simulink model "c63_cylinder_blowdown_ref"  (R2026a)
settings: Solver=ode4  StopTime=S12_BlowdownStopTimeS  FixedStep=1e-6
model workspace (MAT data in the model file):
  S12_BlowdownStopTimeS = Simulink.Parameter
  S12_BlowdownStopTimeS.Value = 0.0266666666667
  S12_BlowdownStopTimeS.Complexity = 'real'
  S12_BlowdownStopTimeS.Dimensions = [1 1]
  S12_BlowdownStopTimeS.Description = 'Run from -180 to +300 deg ATDC'
  S12_BlowdownStopTimeS.DataType = 'auto'
  S12_BlowdownStopTimeS.DocUnits = 's'
  S12_BurnedCpJkgK = Simulink.Parameter
  S12_BurnedCpJkgK.Value = [1075.46244927 1100.31766319 1127.88587263 1157.95433687 1189.74992272 1221.93910449 1252.627964 1279.36219058 1303.34621886 1325.27401636 1345.29919881 1363.55240895 1380.1594629 1395.24135019 1408.91423372 1421.28944978 1432.47350805 1442.56809158 1451.67005684 1459.87143365 1467.25942525 1473.91640823 1479.91993261 1485.34272177 1490.25267247 1494.71285488 1498.78151253 1502.51206237 1505.9530947 1509.14837323 1512.13683507 1514.95259067 1517.62492391]
  S12_BurnedCpJkgK.Complexity = 'real'
  S12_BurnedCpJkgK.Dimensions = [1 33]
  S12_BurnedCpJkgK.Description = 'Derived from NASA species polynomial mixture tables'
  S12_BurnedCpJkgK.DataType = 'auto'
  S12_BurnedCpJkgK.DocUnits = 'J/(kg*K)'
  S12_BurnedGasConstantJkgK = Simulink.Parameter
  S12_BurnedGasConstantJkgK.Value = 290.645082378
  S12_BurnedGasConstantJkgK.Complexity = 'real'
  S12_BurnedGasConstantJkgK.Dimensions = [1 1]
  S12_BurnedGasConstantJkgK.Description = 'Derived from NASA species polynomial mixture tables'
  S12_BurnedGasConstantJkgK.DataType = 'auto'
  S12_BurnedGasConstantJkgK.DocUnits = 'J/(kg*K)'
  S12_C63_BoreM = Simulink.Parameter
  S12_C63_BoreM.Value = 0.1022
  S12_C63_BoreM.Complexity = 'real'
  S12_C63_BoreM.Dimensions = [1 1]
  S12_C63_BoreM.Description = 'Grade A M156.985 bore'
  S12_C63_BoreM.DataType = 'auto'
  S12_C63_BoreM.DocUnits = 'm'
  S12_C63_CompressionRatio = Simulink.Parameter
  S12_C63_CompressionRatio.Value = 11.3
  S12_C63_CompressionRatio.Complexity = 'real'
  S12_C63_CompressionRatio.Dimensions = [1 1]
  S12_C63_CompressionRatio.Description = 'Grade A M156.985 compression ratio'
  S12_C63_CompressionRatio.DataType = 'auto'
  S12_C63_RodLengthM = Simulink.Parameter
  S12_C63_RodLengthM.Value = 0.1455
  S12_C63_RodLengthM.Complexity = 'real'
  S12_C63_RodLengthM.Dimensions = [1 1]
  S12_C63_RodLengthM.Description = 'Grade D identification initial value'
  S12_C63_RodLengthM.DataType = 'auto'
  S12_C63_RodLengthM.DocUnits = 'm'
  S12_C63_StrokeM = Simulink.Parameter
  S12_C63_StrokeM.Value = 0.0946
  S12_C63_StrokeM.Complexity = 'real'
  S12_C63_StrokeM.Dimensions = [1 1]
  S12_C63_StrokeM.Description = 'Grade A M156.985 stroke'
  S12_C63_StrokeM.DataType = 'auto'
  S12_C63_StrokeM.DocUnits = 'm'
  S12_CrankDegPerSecond = Simulink.Parameter
  S12_CrankDegPerSecond.Value = 18000
  S12_CrankDegPerSecond.Complexity = 'real'
  S12_CrankDegPerSecond.Dimensions = [1 1]
  S12_CrankDegPerSecond.Description = 'Derived crank speed'
  S12_CrankDegPerSecond.DataType = 'auto'
  S12_CrankDegPerSecond.DocUnits = 'deg/s'
  S12_DownstreamPressurePa = Simulink.Parameter
  S12_DownstreamPressurePa.Value = 101325
  S12_DownstreamPressurePa.Complexity = 'real'
  S12_DownstreamPressurePa.Dimensions = [1 1]
  S12_DownstreamPressurePa.Description = 'Reference exhaust manifold pressure'
  S12_DownstreamPressurePa.DataType = 'auto'
  S12_DownstreamPressurePa.DocUnits = 'Pa'
  S12_EngineRPM = Simulink.Parameter
  S12_EngineRPM.Value = 3000
  S12_EngineRPM.Complexity = 'real'
  S12_EngineRPM.Dimensions = [1 1]
  S12_EngineRPM.Description = 'Reference operating point'
  S12_EngineRPM.DataType = 'auto'
  S12_EngineRPM.DocUnits = 'rpm'
  S12_EvoDegATDC = Simulink.Parameter
  S12_EvoDegATDC.Value = 130
  S12_EvoDegATDC.Complexity = 'real'
  S12_EvoDegATDC.Dimensions = [1 1]
  S12_EvoDegATDC.Description = 'Grade D EVO initial value'
  S12_EvoDegATDC.DataType = 'auto'
  S12_EvoDegATDC.DocUnits = 'deg'
  S12_ExhaustDurationDeg = Simulink.Parameter
  S12_ExhaustDurationDeg.Value = 220
  S12_ExhaustDurationDeg.Complexity = 'real'
  S12_ExhaustDurationDeg.Dimensions = [1 1]
  S12_ExhaustDurationDeg.Description = 'Grade D exhaust duration'
  S12_ExhaustDurationDeg.DataType = 'auto'
  S12_ExhaustDurationDeg.DocUnits = 'deg'
  S12_ExhaustPortEffectiveAreaM2 = Simulink.Parameter
  S12_ExhaustPortEffectiveAreaM2.Value = 0.0012
  S12_ExhaustPortEffectiveAreaM2.Complexity = 'real'
  S12_ExhaustPortEffectiveAreaM2.Dimensions = [1 1]
  S12_ExhaustPortEffectiveAreaM2.Description = 'Grade D effective port cap'
  S12_ExhaustPortEffectiveAreaM2.DataType = 'auto'
  S12_ExhaustPortEffectiveAreaM2.DocUnits = 'm^2'
  S12_ExhaustValveCount = Simulink.Parameter
  S12_ExhaustValveCount.Value = 2
  S12_ExhaustValveCount.Complexity = 'real'
  S12_ExhaustValveCount.Dimensions = [1 1]
  S12_ExhaustValveCount.Description = 'Two exhaust valves per cylinder'
  S12_ExhaustValveCount.DataType = 'auto'
  S12_ExhaustValveDiameterM = Simulink.Parameter
  S12_ExhaustValveDiameterM.Value = 0.034
  S12_ExhaustValveDiameterM.Complexity = 'real'
  S12_ExhaustValveDiameterM.Dimensions = [1 1]
  S12_ExhaustValveDiameterM.Description = 'Grade C exhaust valve diameter'
  S12_ExhaustValveDiameterM.DataType = 'auto'
  S12_ExhaustValveDiameterM.DocUnits = 'm'
  S12_ExhaustValveLiftM = Simulink.Parameter
  S12_ExhaustValveLiftM.Value = 0.0105
  S12_ExhaustValveLiftM.Complexity = 'real'
  S12_ExhaustValveLiftM.Dimensions = [1 1]
  S12_ExhaustValveLiftM.Description = 'Grade D valve lift initial value'
  S12_ExhaustValveLiftM.DataType = 'auto'
  S12_ExhaustValveLiftM.DocUnits = 'm'
  S12_FreshCpJkgK = Simulink.Parameter
  S12_FreshCpJkgK.Value = [1011.44586028 1020.85335446 1036.72053362 1057.5147036 1081.40452476 1106.26001208 1129.65253503 1148.85481767 1165.4715059 1180.60214876 1194.36500843 1206.87270224 1218.23218208 1228.54473438 1237.90598016 1246.40587499 1254.12870897 1261.15310681 1267.55202774 1273.39276557 1278.73694867 1283.64053995 1288.1538369 1292.32147156 1296.18241054 1299.76995499 1303.11174065 1306.22973779 1309.14025125 1311.85392043 1314.37571931 1316.70495638 1318.83527475]
  S12_FreshCpJkgK.Complexity = 'real'
  S12_FreshCpJkgK.Dimensions = [1 33]
  S12_FreshCpJkgK.Description = 'Derived from NASA species polynomial mixture tables'
  S12_FreshCpJkgK.DataType = 'auto'
  S12_FreshCpJkgK.DocUnits = 'J/(kg*K)'
  S12_FreshGasConstantJkgK = Simulink.Parameter
  S12_FreshGasConstantJkgK.Value = 288.19294148
  S12_FreshGasConstantJkgK.Complexity = 'real'
  S12_FreshGasConstantJkgK.Dimensions = [1 1]
  S12_FreshGasConstantJkgK.Description = 'Derived from NASA species polynomial mixture tables'
  S12_FreshGasConstantJkgK.DataType = 'auto'
  S12_FreshGasConstantJkgK.DocUnits = 'J/(kg*K)'
  S12_HeatPerCycleJ = Simulink.Parameter
  S12_HeatPerCycleJ.Value = 2100
  S12_HeatPerCycleJ.Complexity = 'real'
  S12_HeatPerCycleJ.Dimensions = [1 1]
  S12_HeatPerCycleJ.Description = 'Grade D heat initial value; identify from IMEP'
  S12_HeatPerCycleJ.DataType = 'auto'
  S12_HeatPerCycleJ.DocUnits = 'J'
  S12_InitialMassKg = Simulink.Parameter
  S12_InitialMassKg.Value = 0.000907075341472
  S12_InitialMassKg.Complexity = 'real'
  S12_InitialMassKg.Dimensions = [1 1]
  S12_InitialMassKg.Description = 'Derived initial trapped mass from pV=mRT'
  S12_InitialMassKg.DataType = 'auto'
  S12_InitialMassKg.DocUnits = 'kg'
  S12_InitialPressurePa = Simulink.Parameter
  S12_InitialPressurePa.Value = 101325
  S12_InitialPressurePa.Complexity = 'real'
  S12_InitialPressurePa.Dimensions = [1 1]
  S12_InitialPressurePa.Description = 'Reference pressure at compression BDC'
  S12_InitialPressurePa.DataType = 'auto'
  S12_InitialPressurePa.DocUnits = 'Pa'
  S12_InitialTemperatureK = Simulink.Parameter
  S12_InitialTemperatureK.Value = 330
  S12_InitialTemperatureK.Complexity = 'real'
  S12_InitialTemperatureK.Dimensions = [1 1]
  S12_InitialTemperatureK.Description = 'Reference temperature at compression BDC'
  S12_InitialTemperatureK.DataType = 'auto'
  S12_InitialTemperatureK.DocUnits = 'K'
  S12_PropertyTemperatureK = Simulink.Parameter
  S12_PropertyTemperatureK.Value = [300 400 500 600 700 800 900 1000 1100 1200 1300 1400 1500 1600 1700 1800 1900 2000 2100 2200 2300 2400 2500 2600 2700 2800 2900 3000 3100 3200 3300 3400 3500]
  S12_PropertyTemperatureK.Complexity = 'real'
  S12_PropertyTemperatureK.Dimensions = [1 33]
  S12_PropertyTemperatureK.Description = 'Derived from NASA species polynomial mixture tables'
  S12_PropertyTemperatureK.DataType = 'auto'
  S12_PropertyTemperatureK.DocUnits = 'K'
  S12_ValveDischargeCoefficient = Simulink.Parameter
  S12_ValveDischargeCoefficient.Value = 0.72
  S12_ValveDischargeCoefficient.Complexity = 'real'
  S12_ValveDischargeCoefficient.Dimensions = [1 1]
  S12_ValveDischargeCoefficient.Description = 'Grade D constant Cd; later replace with Cd(lift)'
  S12_ValveDischargeCoefficient.DataType = 'auto'
  S12_WallTemperatureK = Simulink.Parameter
  S12_WallTemperatureK.Value = 430
  S12_WallTemperatureK.Complexity = 'real'
  S12_WallTemperatureK.Dimensions = [1 1]
  S12_WallTemperatureK.Description = 'Reference warm wall'
  S12_WallTemperatureK.DataType = 'auto'
  S12_WallTemperatureK.DocUnits = 'K'
  S12_WiebeA = Simulink.Parameter
  S12_WiebeA.Value = 6.9
  S12_WiebeA.Complexity = 'real'
  S12_WiebeA.Dimensions = [1 1]
  S12_WiebeA.Description = 'Wiebe completion parameter'
  S12_WiebeA.DataType = 'auto'
  S12_WiebeDurationDeg = Simulink.Parameter
  S12_WiebeDurationDeg.Value = 50
  S12_WiebeDurationDeg.Complexity = 'real'
  S12_WiebeDurationDeg.Dimensions = [1 1]
  S12_WiebeDurationDeg.Description = 'Grade D combustion duration initial value'
  S12_WiebeDurationDeg.DataType = 'auto'
  S12_WiebeDurationDeg.DocUnits = 'deg'
  S12_WiebeM = Simulink.Parameter
  S12_WiebeM.Value = 2
  S12_WiebeM.Complexity = 'real'
  S12_WiebeM.Dimensions = [1 1]
  S12_WiebeM.Description = 'Grade D Wiebe shape'
  S12_WiebeM.DataType = 'auto'
  S12_WiebeStartDeg = Simulink.Parameter
  S12_WiebeStartDeg.Value = -20
  S12_WiebeStartDeg.Complexity = 'real'
  S12_WiebeStartDeg.Dimensions = [1 1]
  S12_WiebeStartDeg.Description = 'Grade D combustion phasing initial value'
  S12_WiebeStartDeg.DataType = 'auto'
  S12_WiebeStartDeg.DocUnits = 'deg'
settings Model: Creator=Jovi  LastModifiedBy=Jovi

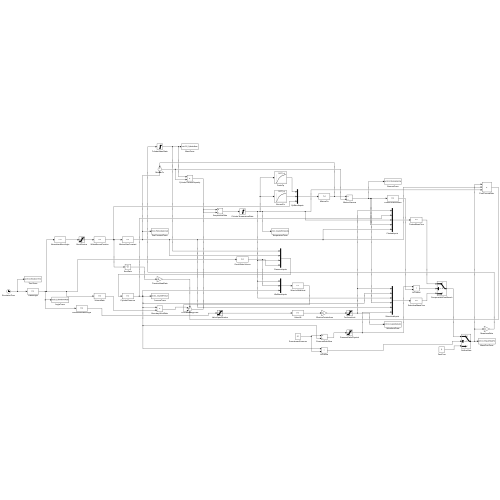
[thumbnail: Simulink's stored preview of the top-level diagram]
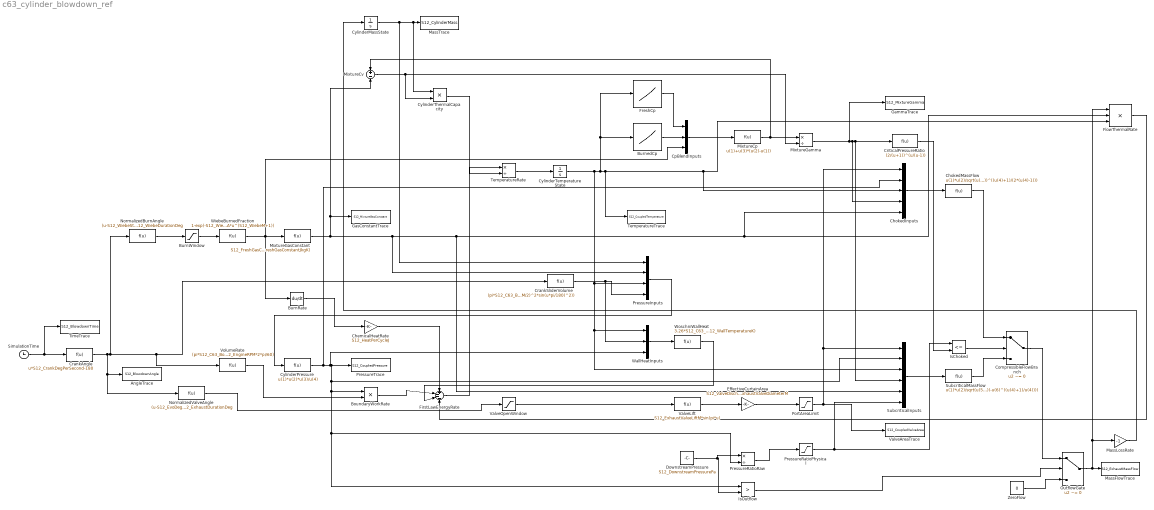
== system c63_cylinder_blowdown_ref ==
  AngleTrace : ToWorkspace  VariableName=S12_BlowdownAngle
      settings: MaxDataPoints=50000
  BoundaryWorkRate : Product
  BurnRate : Derivative
  BurnWindow : Saturate  UpperLimit=1  LowerLimit=0
  BurnedCp : Lookup_n-D  NumberOfTableDimensions=1  BreakpointsForDimension1=S12_PropertyTemperatureK  Table=S12_BurnedCpJkgK  InternalRulePriority=Speed  RndMeth=Simplest
  ChemicalHeatRate : Gain  Gain=S12_HeatPerCycleJ
  ChokedInputs : Mux  Inputs=5
  ChokedMassFlow : Fcn  Expr=u(1)*u(2)/sqrt(u(5)*u(3))*sqrt(u(4))*(2/(u(4)+1))^((u(4)+1)/(2*(u(4)-1)))
  CompressibleFlowBranch : Switch  Criteria=u2 ~= 0  Threshold=0.5
  CpBlendInputs : Mux  Inputs=3
  CrankAngle : Fcn  Expr=u*S12_CrankDegPerSecond-180
  CrankSliderVolume : Fcn  Expr=(pi*S12_C63_BoreM^2*S12_C63_StrokeM/4)/(S12_C63_CompressionRatio-1)+(pi*S12_C63_BoreM^2/4)*((S12_C63_StrokeM/2)*(1-cos(u*pi/180))+S12_C63_RodLengthM-sqrt(S12_C63_RodLengthM^2-(S12_C63_StrokeM/2)^2*sin(u*pi/180)^2))
  CriticalPressureRatio : Fcn  Expr=(2/(u+1))^(u/(u-1))
  CylinderMassState : Integrator  InitialCondition=S12_InitialMassKg  LimitOutput=on  LowerSaturationLimit=1e-8
  CylinderPressure : Fcn  Expr=u(1)*u(2)*u(3)/u(4)
  CylinderTemperatureState : Integrator  InitialCondition=S12_InitialTemperatureK  LimitOutput=on  UpperSaturationLimit=5000  LowerSaturationLimit=250
  CylinderThermalCapacity : Product
  DownstreamPressure : Constant  Value=S12_DownstreamPressurePa
  EffectiveCurtainArea : Gain  Gain=S12_ValveDischargeCoefficient*S12_ExhaustValveCount*pi*S12_ExhaustValveDiameterM
  FirstLawEnergyRate : Sum  Inputs=+---
  FlowThermalRate : Product  Inputs=***
  FreshCp : Lookup_n-D  NumberOfTableDimensions=1  BreakpointsForDimension1=S12_PropertyTemperatureK  Table=S12_FreshCpJkgK  InternalRulePriority=Speed  RndMeth=Simplest
  GammaTrace : ToWorkspace  VariableName=S12_MixtureGamma
      settings: MaxDataPoints=50000
  GasConstantTrace : ToWorkspace  VariableName=S12_MixtureGasConstant
      settings: MaxDataPoints=50000
  IsChoked : RelationalOperator  Operator=<=
  IsOutflow : RelationalOperator  Operator=>
  MassFlowTrace : ToWorkspace  VariableName=S12_ExhaustMassFlow
      settings: MaxDataPoints=50000
  MassLossRate : Gain  Gain=-1
  MassTrace : ToWorkspace  VariableName=S12_CylinderMass
      settings: MaxDataPoints=50000
  MixtureCp : Fcn  Expr=u(1)+u(3)*(u(2)-u(1))
  MixtureCv : Sum  Inputs=+-
  MixtureGamma : Product  Inputs=*/
  MixtureGasConstant : Fcn  Expr=S12_FreshGasConstantJkgK+u*(S12_BurnedGasConstantJkgK-S12_FreshGasConstantJkgK)
  NormalizedBurnAngle : Fcn  Expr=(u-S12_WiebeStartDeg)/S12_WiebeDurationDeg
  NormalizedValveAngle : Fcn  Expr=(u-S12_EvoDegATDC)/S12_ExhaustDurationDeg
  OutflowGate : Switch  Criteria=u2 ~= 0  Threshold=0.5
  PortAreaLimit : Saturate  UpperLimit=S12_ExhaustPortEffectiveAreaM2  LowerLimit=0
  PressureInputs : Mux
  PressureRatioPhysical : Saturate  UpperLimit=1  LowerLimit=0
  PressureRatioRaw : Product  Inputs=*/
  PressureTrace : ToWorkspace  VariableName=S12_CoupledPressure
      settings: MaxDataPoints=50000
  SimulationTime : Clock
  SubcriticalInputs : Mux  Inputs=6
  SubcriticalMassFlow : Fcn  Expr=u(1)*u(2)/sqrt(u(5)*u(3))*sqrt(2*u(4)/(u(4)-1)*(u(6)^(2/u(4))-u(6)^((u(4)+1)/u(4))))
  TemperatureRate : Product  Inputs=*/
  TemperatureTrace : ToWorkspace  VariableName=S12_CoupledTemperature
      settings: MaxDataPoints=50000
  TimeTrace : ToWorkspace  VariableName=S12_BlowdownTime
      settings: MaxDataPoints=50000
  ValveAreaTrace : ToWorkspace  VariableName=S12_CoupledValveArea
      settings: MaxDataPoints=50000
  ValveLift : Fcn  Expr=S12_ExhaustValveLiftM*sin(pi*u)
  ValveOpenWindow : Saturate  UpperLimit=1  LowerLimit=0
  VolumeRate : Fcn  Expr=(pi*S12_C63_BoreM^2/4)*((S12_C63_StrokeM/2)*sin(u*pi/180)+(S12_C63_StrokeM/2)^2*sin(u*pi/180)*cos(u*pi/180)/sqrt(S12_C63_RodLengthM^2-(S12_C63_StrokeM/2)^2*sin(u*pi/180)^2))*(S12_EngineRPM*2*pi/60)
  WallHeatInputs : Mux  Inputs=3
  WiebeBurnedFraction : Fcn  Expr=1-exp(-S12_WiebeA*u^(S12_WiebeM+1))
  WoschniWallHeat : Fcn  Expr=3.26*S12_C63_BoreM^(-0.2)*(u(3)/1000)^0.8*u(1)^(-0.55)*(2.28*(2*S12_C63_StrokeM*S12_EngineRPM/60))^0.8*(2*pi*S12_C63_BoreM^2/4+pi*S12_C63_BoreM*((u(2)-(pi*S12_C63_BoreM^2*S12_C63_StrokeM/4)/(S12_C63_CompressionRatio-1))/(pi*S12_C63_BoreM^2/4)))*(u(1)-S12_WallTemperatureK)
  ZeroFlow : Constant  Value=0
  wires:
  TemperatureRate/1 -> CylinderTemperatureState/1
  CylinderThermalCapacity/1 -> TemperatureRate/2
  FirstLawEnergyRate/1 -> TemperatureRate/1
  FlowThermalRate/1 -> FirstLawEnergyRate/4
  WoschniWallHeat/1 -> FirstLawEnergyRate/3
  BoundaryWorkRate/1 -> FirstLawEnergyRate/2
  ChemicalHeatRate/1 -> FirstLawEnergyRate/1
  VolumeRate/1 -> BoundaryWorkRate/2
  WallHeatInputs/1 -> WoschniWallHeat/1
  MassLossRate/1 -> CylinderMassState/1
  OutflowGate/1 -> MassLossRate/1, FlowThermalRate/1, MassFlowTrace/1
  ZeroFlow/1 -> OutflowGate/3
  IsOutflow/1 -> OutflowGate/2
  CompressibleFlowBranch/1 -> OutflowGate/1
  SubcriticalMassFlow/1 -> CompressibleFlowBranch/3
  IsChoked/1 -> CompressibleFlowBranch/2
  ChokedMassFlow/1 -> CompressibleFlowBranch/1
  SubcriticalInputs/1 -> SubcriticalMassFlow/1
  ChokedInputs/1 -> ChokedMassFlow/1
  PortAreaLimit/1 -> ChokedInputs/1, SubcriticalInputs/1, ValveAreaTrace/1
  CriticalPressureRatio/1 -> IsChoked/2
  PressureRatioPhysical/1 -> IsChoked/1, SubcriticalInputs/6
  MixtureGamma/1 -> CriticalPressureRatio/1, SubcriticalInputs/4, ChokedInputs/4, GammaTrace/1
  PressureRatioRaw/1 -> PressureRatioPhysical/1
  CylinderPressure/1 -> PressureRatioRaw/2, IsOutflow/1, BoundaryWorkRate/1, SubcriticalInputs/2, PressureTrace/1, WallHeatInputs/3, ChokedInputs/2
  DownstreamPressure/1 -> PressureRatioRaw/1, IsOutflow/2
  EffectiveCurtainArea/1 -> PortAreaLimit/1
  ValveLift/1 -> EffectiveCurtainArea/1
  ValveOpenWindow/1 -> ValveLift/1
  NormalizedValveAngle/1 -> ValveOpenWindow/1
  PressureInputs/1 -> CylinderPressure/1
  CrankSliderVolume/1 -> PressureInputs/4, WallHeatInputs/2
  CylinderMassState/1 -> CylinderThermalCapacity/1, MassTrace/1, PressureInputs/1
  MixtureCv/1 -> MixtureGamma/2, CylinderThermalCapacity/2
  MixtureGasConstant/1 -> FlowThermalRate/2, ChokedInputs/5, SubcriticalInputs/5, PressureInputs/2, MixtureCv/2, GasConstantTrace/1
  MixtureCp/1 -> MixtureCv/1, MixtureGamma/1
  CpBlendInputs/1 -> MixtureCp/1
  BurnedCp/1 -> CpBlendInputs/2
  FreshCp/1 -> CpBlendInputs/1
  CylinderTemperatureState/1 -> WallHeatInputs/1, SubcriticalInputs/3, PressureInputs/3, ChokedInputs/3, FlowThermalRate/3, TemperatureTrace/1, FreshCp/1, BurnedCp/1
  BurnRate/1 -> ChemicalHeatRate/1
  WiebeBurnedFraction/1 -> BurnRate/1, MixtureGasConstant/1, CpBlendInputs/3
  BurnWindow/1 -> WiebeBurnedFraction/1
  NormalizedBurnAngle/1 -> BurnWindow/1
  CrankAngle/1 -> NormalizedValveAngle/1, AngleTrace/1, CrankSliderVolume/1, VolumeRate/1, NormalizedBurnAngle/1
  SimulationTime/1 -> CrankAngle/1, TimeTrace/1
